simulink model "robot_4DOF"  (Simulink 7.3)
settings: Solver=ode45  StartTime=0.0  StopTime=10.0  RelTol=1e-3
libraries: dspinverses x1
settings Model: Creator=arash  LastModifiedBy=arash  TunableVars=I1,I2,I3,I4,Ixx1,Ixx2,Ixx3,Ixx4,Iyy1,Iyy2,Iyy3,Iyy4,Izz1,Izz2,Izz3,Izz4,Kd,Ki,Kp,Ts,c1,c2,c3,c4,g,l1,l2,l3,l4,m1,m2,m3,m4,statesint,tauin,tout,yout  TunableVarsStorageClass=Auto,Auto,Auto,Auto,Auto,Auto,Auto,Auto,Auto,Auto,Auto,Auto,Auto,Auto,Auto,Auto,Auto,Auto,Auto,Auto,Auto,Auto,Auto,Auto,Auto,Auto,Auto,Auto,Auto,Auto,Auto,Auto,Auto,Auto,Auto,Auto,Auto  TunableVarsTypeQualifier=,,,,,,,,,,,,,,,,,,,,,,,,,,,,,,,,,,,,
settings OptimizationCC: InlineParams=on

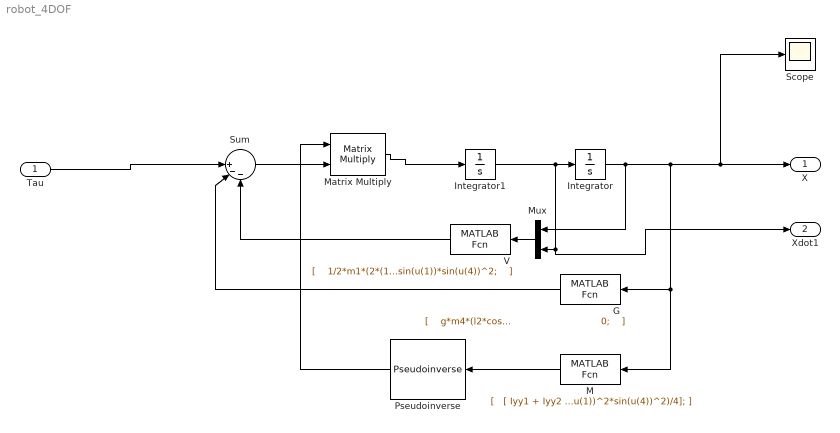
== system robot_4DOF ==
  Tau : Inport  OutDataType=fixdt(1, 16)  OutScaling=2^0
  G : MATLABFcn  MATLABFcn=|  OutputDimensions=4  OutputSignalType=real  Output1D=off
      | [
      |  
      |  g*m4*(l2*cos(u(1) + u(2)) + l1*cos(u(1)) + 1/2*l3*cos(u(1) + u(2) + u(3))) + g*m3*(1/2*l2*cos(u(1) + u(2)) + l1*cos(u(1))) + 1/2*g*l1*m2*cos(u(1));
      |                                                          g*m4*(l2*cos(u(1) + u(2)) + 1/2*l3*cos(u(1) + u(2) + u(3))) + 1/2*g*l2*m3*cos(u(1) + u(2));
      |                                                                                                                 1/2*g*l3*m4*cos(u(1) + u(2) + u(3));
      |                                                                                                                                                   0;
      |  
      |  ]
  Integrator : Integrator
  Integrator1 : Integrator
  M : MATLABFcn  MATLABFcn=|  OutputDimensions=[4 4]  OutputSignalType=real  Output1D=off
      | [
      |  
      | [ Iyy1 + Iyy2 + 1.0*Iyy3 + (m3*(2*(1.0*l2*sin(u(1) + u(2)) + l1*sin(u(1)) + 0.5*l3*sin(u(1) + u(2) + u(3)))*(l2*sin(u(1) + u(2)) + l1*sin(u(1)) + (l3*sin(u(1) + u(2) + u(3)))/2)*cos(u(4))^2 + 2*(1.0*l2*sin(u(1) + u(2)) + l1*sin(u(1)) + 0.5*l3*sin(u(1) + u(2) + u(3)))*(l2*sin(u(1) + u(2)) + l1*sin(u(1)) + (l3*sin(u(1) + u(2) + u(3)))/2)*sin(u(4))^2 + 2*(l2*cos(u(1) + u(2)) + l1*cos(u(1)) + (l3*cos(u(1) + u(2) + u(3)))/2)*(1.0*l2*cos(u(1) + u(2)) + l1*cos(u(1)) + 0.5*l3*cos(u(1) + u(2) + u(3)))))/2 + (l1^2*m1)/4 + (m2*(2*((l2*sin(u(1) + u(2)))/2 + l1*sin(u(1)))*(0.5*l2*sin(u(1) + u(2)) + l1*sin(u(1)))*cos(u(4))^2 + 2*((l2*sin(u(1) + u(2)))/2 + l1*sin(u(1)))*(0.5*l2*sin(u(1) + u(2)) + l1*sin(u(1)))*sin(u(4))^2 + 2*((l2*cos(u(1) + u(2)))/2 + l1*cos(u(1)))*(0.5*l2*cos(u(1) + u(2)) + l1*cos(u(1)))))/2, Iyy2 + 1.0*Iyy3 + (m3*(2*(1.0*l2*sin(u(1) + u(2)) + 0.5*l3*sin(u(1) + u(2) + u(3)))*(l2*sin(u(1) + u(2)) + l1*sin(u(1)) + (l3*sin(u(1) + u(2) + u(3)))/2)*cos(u(4))^2 + 2*(1.0*l2*sin(u(1) + u(2)) + 0.5*l3*sin(u(1) + u(2) + u(3)))*(l2*sin(u(1) + u(2)) + l1*sin(u(1)) + (l3*sin(u(1) + u(2) + u(3)))/2)*sin(u(4))^2 + 2*(1.0*l2*cos(u(1) + u(2)) + 0.5*l3*cos(u(1) + u(2) + u(3)))*(l2*cos(u(1) + u(2)) + l1*cos(u(1)) + (l3*cos(u(1) + u(2) + u(3)))/2)))/2 + (m2*(1.0*l2*sin(u(1) + u(2))*((l2*sin(u(1) + u(2)))/2 + l1*sin(u(1)))*cos(u(4))^2 + 1.0*l2*sin(u(1) + u(2))*((l2*sin(u(1) + u(2)))/2 + l1*sin(u(1)))*sin(u(4))^2 + 1.0*l2*cos(u(1) + u(2))*((l2*cos(u(1) + u(2)))/2 + l1*cos(u(1)))))/2, 1.0*Iyy3 + (m3*(1.0*l3*sin(u(1) + u(2) + u(3))*(l2*sin(u(1) + u(2)) + l1*sin(u(1)) + (l3*sin(u(1) + u(2) + u(3)))/2)*cos(u(4))^2 + 1.0*l3*sin(u(1) + u(2) + u(3))*(l2*sin(u(1) + u(2)) + l1*sin(u(1)) + (l3*sin(u(1) + u(2) + u(3)))/2)*sin(u(4))^2 + 1.0*l3*cos(u(1) + u(2) + u(3))*(l2*cos(u(1) + u(2)) + l1*cos(u(1)) + (l3*cos(u(1) + u(2) + u(3)))/2)))/2,                                                                                                                                                                                                                                                                                                                                                                                                                                                                                                                                                                                    0];
      | [                                                                                                                                                                                                                                                                                                                                                                                                                                                                                                                                                                                                                                                                                 Iyy2 + Iyy3 + (l2^2*m2)/4 + l2^2*m3 + (l3^2*m3)/4 + (l1*l3*m3*cos(u(2) + u(3)))/2 + (l1*l2*m2*cos(u(2)))/2 + l1*l2*m3*cos(u(2)) + l2*l3*m3*cos(u(3)),                                                                                                                                                                                                                                                                                                                                                                                                                                                                                                                                                                                                                                    Iyy2 + Iyy3 + (l2^2*m2)/4 + l2^2*m3 + (l3^2*m3)/4 + l2*l3*m3*cos(u(3)),                                                                                                                                                                                                                                                                                                                    (m3*l3^2)/4 + (l2*m3*cos(u(3))*l3)/2 + Iyy3,                                                                                                                                                                                                                                                                                                                                                                                                                                                                                                                                                                                    0];
      | [                                                                                                                                                                                                                                                                                                                                                                                                                                                                                                                                                                                                                                                                                                                                                          Iyy3 + (l3^2*m3)/4 + (l1*l3*m3*cos(u(2) + u(3)))/2 + (l2*l3*m3*cos(u(3)))/2,                                                                                                                                                                                                                                                                                                                                                                                                                                                                                                                                                                                                                                                               (m3*l3^2)/4 + (l2*m3*cos(u(3))*l3)/2 + Iyy3,                                                                                                                                                                                                                                                                                                                                             (m3*l3^2)/4 + Iyy3,                                                                                                                                                                                                                                                                                                                                                                                                                                                                                                                                                                                    0];
      | [                                                                                                                                                                                                                                                                                                                                                                                                                                                                                                                                                                                                                                                                                                                                                                                                                                    0,                                                                                                                                                                                                                                                                                                                                                                                                                                                                                                                                                                                                                                                                                                         0,                                                                                                                                                                                                                                                                                                                                                              0, I4 - Izz2*(cos(u(1) + u(2))^2 - 1) + (m2*(2*cos(u(4))^2*((l2*cos(u(1) + u(2)))/2 + l1*cos(u(1)))^2 + 2*sin(u(4))^2*((l2*cos(u(1) + u(2)))/2 + l1*cos(u(1)))^2))/2 + Ixx3*cos(u(1) + u(2) + u(3))^2 - Izz1*(cos(u(1))^2 - 1) - Izz3*(cos(u(1) + u(2) + u(3))^2 - 1) + Ixx2*cos(u(1) + u(2))^2 + Ixx1*cos(u(1))^2 + (m3*(2*cos(u(4))^2*(l2*cos(u(1) + u(2)) + l1*cos(u(1)) + (l3*cos(u(1) + u(2) + u(3)))/2)^2 + 2*sin(u(4))^2*(l2*cos(u(1) + u(2)) + l1*cos(u(1)) + (l3*cos(u(1) + u(2) + u(3)))/2)^2))/2 + (l1^2*m1*cos(u(1))^2*cos(u(4))^2)/4 + (l1^2*m1*cos(u(1))^2*sin(u(4))^2)/4];
      | ]
  Matrix Multiply : Product  Multiplication=Matrix(*)  OutDataType=sfix(16)  OutScaling=2^0
  Mux : Mux  Inputs=2
  Pseudoinverse : dspinverses/Pseudoinverse  wanterr=off
  Scope : Scope
      settings: YMin=-2.75  YMax=0.25
  Sum : Sum  Inputs=||+--  OutDataType=fixdt(1, 16)  OutScaling=2^0
  V : MATLABFcn  MATLABFcn=|  OutputDimensions=4  OutputSignalType=real  Output1D=off
      | [
      |  
      |  1/2*m1*(2*(1/2*l1*u(8)*sin(u(1))*sin(u(4)) - 1/2*l1*u(5)*cos(u(1))*cos(u(4)))*(1/2*l1*u(5)*cos(u(4))*sin(u(1)) + 1/2*l1*u(8)*cos(u(1))*sin(u(4))) - 2*(1/2*l1*u(5)*sin(u(1))*sin(u(4)) - 1/2*l1*u(8)*cos(u(1))*cos(u(4)))*(1/2*l1*u(5)*cos(u(1))*sin(u(4)) + 1/2*l1*u(8)*cos(u(4))*sin(u(1))) + 1/2*l1^2*u(5)^2*cos(u(1))*sin(u(1))) + 1/2*m2*(2*sin(u(4))*(1/2*l2*sin(u(1) + u(2)) + l1*sin(u(1)))*(sin(u(4))*(1/2*l2*cos(u(1) + u(2)) + l1*cos(u(1)))*u(8)^2 + 2*cos(u(4))*(l1*u(5)*sin(u(1)) + 1/2*l2*sin(u(1) + u(2))*(u(5) + u(6)))*u(8) + sin(u(4))*(1/2*l2*cos(u(1) + u(2))*(u(5) + u(6))^2 + l1*u(5)^2*cos(u(1)))) - 2*(1/2*l2*sin(u(1) + u(2))*(u(5) + u(6))^2 + l1*u(5)^2*sin(u(1)))*(1/2*l2*cos(u(1) + u(2)) + l1*cos(u(1))) - 2*(l1*u(5)*cos(u(1)) + 1/2*l2*cos(u(1) + u(2))*(u(5) + u(6)))*(l1*u(5)*sin(u(1)) + 1/2*l2*sin(u(1) + u(2))*(u(5) + u(6))) + 2*cos(u(4))*(cos(u(4))*(l1*u(5)*sin(u(1)) + 1/2*l2*sin(u(1) + u(2))*(u(5) + u(6))) + u(8)*sin(u(4))*(1/2*l2*cos(u(1) + u(2)) + l1*cos(u(1))))*(l1*u(5)*cos(u(1)) + 1/2*l2*cos(u(1) + u(2))*(u(5) + u(6))) + 2*sin(u(4))*(sin(u(4))*(l1*u(5)*sin(u(1)) + 1/2*l2*sin(u(1) + u(2))*(u(5) + u(6))) - u(8)*cos(u(4))*(1/2*l2*cos(u(1) + u(2)) + l1*cos(u(1))))*(l1*u(5)*cos(u(1)) + 1/2*l2*cos(u(1) + u(2))*(u(5) + u(6))) + 2*cos(u(4))*(1/2*l2*sin(u(1) + u(2)) + l1*sin(u(1)))*(cos(u(4))*(1/2*l2*cos(u(1) + u(2)) + l1*cos(u(1)))*u(8)^2 - 2*sin(u(4))*(l1*u(5)*sin(u(1)) + 1/2*l2*sin(u(1) + u(2))*(u(5) + u(6)))*u(8) + cos(u(4))*(1/2*l2*cos(u(1) + u(2))*(u(5) + u(6))^2 + l1*u(5)^2*cos(u(1)))) + 2*u(8)*cos(u(4))*(sin(u(4))*(l1*u(5)*sin(u(1)) + 1/2*l2*sin(u(1) + u(2))*(u(5) + u(6))) - u(8)*cos(u(4))*(1/2*l2*cos(u(1) + u(2)) + l1*cos(u(1))))*(1/2*l2*sin(u(1) + u(2)) + l1*sin(u(1))) - 2*u(8)*sin(u(4))*(cos(u(4))*(l1*u(5)*sin(u(1)) + 1/2*l2*sin(u(1) + u(2))*(u(5) + u(6))) + u(8)*sin(u(4))*(1/2*l2*cos(u(1) + u(2)) + l1*cos(u(1))))*(1/2*l2*sin(u(1) + u(2)) + l1*sin(u(1)))) + c1*u(5) - 1/2*m3*(2*(sin(u(4))*(l1*u(5)*cos(u(1)) + 1/2*l3*cos(u(1) + u(2) + u(3))*(u(5) + u(6) + u(7)) + l2*cos(u(1) + u(2))*(u(5) + u(6))) + u(8)*cos(u(4))*(l2*sin(u(1) + u(2)) + l1*sin(u(1)) + 1/2*l3*sin(u(1) + u(2) + u(3))))*(sin(u(4))*(l1*u(5)*sin(u(1)) + 1/2*l3*sin(u(1) + u(2) + u(3))*(u(5) + u(6) + u(7)) + l2*sin(u(1) + u(2))*(u(5) + u(6))) - u(8)*cos(u(4))*(l2*cos(u(1) + u(2)) + l1*cos(u(1)) + 1/2*l3*cos(u(1) + u(2) + u(3)))) - 2*(l1*u(5)*sin(u(1)) + 1/2*l3*sin(u(1) + u(2) + u(3))*(u(5) + u(6) + u(7)) + l2*sin(u(1) + u(2))*(u(5) + u(6)))*(l1*u(5)*cos(u(1)) + 1/2*l3*cos(u(1) + u(2) + u(3))*(u(5) + u(6) + u(7)) + l2*cos(u(1) + u(2))*(u(5) + u(6))) + 2*(cos(u(4))*(l1*u(5)*sin(u(1)) + 1/2*l3*sin(u(1) + u(2) + u(3))*(u(5) + u(6) + u(7)) + l2*sin(u(1) + u(2))*(u(5) + u(6))) + u(8)*sin(u(4))*(l2*cos(u(1) + u(2)) + l1*cos(u(1)) + 1/2*l3*cos(u(1) + u(2) + u(3))))*(cos(u(4))*(l1*u(5)*cos(u(1)) + 1/2*l3*cos(u(1) + u(2) + u(3))*(u(5) + u(6) + u(7)) + l2*cos(u(1) + u(2))*(u(5) + u(6))) - u(8)*sin(u(4))*(l2*sin(u(1) + u(2)) + l1*sin(u(1)) + 1/2*l3*sin(u(1) + u(2) + u(3))))) - 1/2*m2*(2*(sin(u(4))*(l1*u(5)*cos(u(1)) + 1/2*l2*cos(u(1) + u(2))*(u(5) + u(6))) + u(8)*cos(u(4))*(1/2*l2*sin(u(1) + u(2)) + l1*sin(u(1))))*(sin(u(4))*(l1*u(5)*sin(u(1)) + 1/2*l2*sin(u(1) + u(2))*(u(5) + u(6))) - u(8)*cos(u(4))*(1/2*l2*cos(u(1) + u(2)) + l1*cos(u(1)))) + 2*(cos(u(4))*(l1*u(5)*sin(u(1)) + 1/2*l2*sin(u(1) + u(2))*(u(5) + u(6))) + u(8)*sin(u(4))*(1/2*l2*cos(u(1) + u(2)) + l1*cos(u(1))))*(cos(u(4))*(l1*u(5)*cos(u(1)) + 1/2*l2*cos(u(1) + u(2))*(u(5) + u(6))) - u(8)*sin(u(4))*(1/2*l2*sin(u(1) + u(2)) + l1*sin(u(1)))) - 2*(l1*u(5)*cos(u(1)) + 1/2*l2*cos(u(1) + u(2))*(u(5) + u(6)))*(l1*u(5)*sin(u(1)) + 1/2*l2*sin(u(1) + u(2))*(u(5) + u(6)))) + 1/2*m3*(2*cos(u(4))*(l2*sin(u(1) + u(2)) + l1*sin(u(1)) + 1/2*l3*sin(u(1) + u(2) + u(3)))*(cos(u(4))*(l2*cos(u(1) + u(2)) + l1*cos(u(1)) + 1/2*l3*cos(u(1) + u(2) + u(3)))*u(8)^2 - 2*sin(u(4))*(l1*u(5)*sin(u(1)) + 1/2*l3*sin(u(1) + u(2) + u(3))*(u(5) + u(6) + u(7)) + l2*sin(u(1) + u(2))*(u(5) + u(6)))*u(8) + cos(u(4))*(1/2*l3*cos(u(1) + u(2) + u(3))*(u(5) + u(6) + u(7))^2 + l2*cos(u(1) + u(2))*(u(5) + u(6))^2 + l1*u(5)^2*cos(u(1)))) - 2*(1/2*l3*sin(u(1) + u(2) + u(3))*(u(5) + u(6) + u(7))^2 + l2*sin(u(1) + u(2))*(u(5) + u(6))^2 + l1*u(5)^2*sin(u(1)))*(l2*cos(u(1) + u(2)) + l1*cos(u(1)) + 1/2*l3*cos(u(1) + u(2) + u(3))) - 2*(l1*u(5)*sin(u(1)) + 1/2*l3*sin(u(1) + u(2) + u(3))*(u(5) + u(6) + u(7)) + l2*sin(u(1) + u(2))*(u(5) + u(6)))*(l1*u(5)*cos(u(1)) + 1/2*l3*cos(u(1) + u(2) + u(3))*(u(5) + u(6) + u(7)) + l2*cos(u(1) + u(2))*(u(5) + u(6))) + 2*sin(u(4))*(l2*sin(u(1) + u(2)) + l1*sin(u(1)) + 1/2*l3*sin(u(1) + u(2) + u(3)))*(sin(u(4))*(l2*cos(u(1) + u(2)) + l1*cos(u(1)) + 1/2*l3*cos(u(1) + u(2) + u(3)))*u(8)^2 + 2*cos(u(4))*(l1*u(5)*sin(u(1)) + 1/2*l3*sin(u(1) + u(2) + u(3))*(u(5) + u(6) + u(7)) + l2*sin(u(1) + u(2))*(u(5) + u(6)))*u(8) + sin(u(4))*(1/2*l3*cos(u(1) + u(2) + u(3))*(u(5) + u(6) + u(7))^2 + l2*cos(u(1) + u(2))*(u(5) + u(6))^2 + l1*u(5)^2*cos(u(1)))) + 2*cos(u(4))*(cos(u(4))*(l1*u(5)*sin(u(1)) + 1/2*l3*sin(u(1) + u(2) + u(3))*(u(5) + u(6) + u(7)) + l2*sin(u(1) + u(2))*(u(5) + u(6))) + u(8)*sin(u(4))*(l2*cos(u(1) + u(2)) + l1*cos(u(1)) + 1/2*l3*cos(u(1) + u(2) + u(3))))*(l1*u(5)*cos(u(1)) + 1/2*l3*cos(u(1) + u(2) + u(3))*(u(5) + u(6) + u(7)) + l2*cos(u(1) + u(2))*(u(5) + u(6))) + 2*sin(u(4))*(sin(u(4))*(l1*u(5)*sin(u(1)) + 1/2*l3*sin(u(1) + u(2) + u(3))*(u(5) + u(6) + u(7)) + l2*sin(u(1) + u(2))*(u(5) + u(6))) - u(8)*cos(u(4))*(l2*cos(u(1) + u(2)) + l1*cos(u(1)) + 1/2*l3*cos(u(1) + u(2) + u(3))))*(l1*u(5)*cos(u(1)) + 1/2*l3*cos(u(1) + u(2) + u(3))*(u(5) + u(6) + u(7)) + l2*cos(u(1) + u(2))*(u(5) + u(6))) + 2*u(8)*cos(u(4))*(sin(u(4))*(l1*u(5)*sin(u(1)) + 1/2*l3*sin(u(1) + u(2) + u(3))*(u(5) + u(6) + u(7)) + l2*sin(u(1) + u(2))*(u(5) + u(6))) - u(8)*cos(u(4))*(l2*cos(u(1) + u(2)) + l1*cos(u(1)) + 1/2*l3*cos(u(1) + u(2) + u(3))))*(l2*sin(u(1) + u(2)) + l1*sin(u(1)) + 1/2*l3*sin(u(1) + u(2) + u(3))) - 2*u(8)*sin(u(4))*(cos(u(4))*(l1*u(5)*sin(u(1)) + 1/2*l3*sin(u(1) + u(2) + u(3))*(u(5) + u(6) + u(7)) + l2*sin(u(1) + u(2))*(u(5) + u(6))) + u(8)*sin(u(4))*(l2*cos(u(1) + u(2)) + l1*cos(u(1)) + 1/2*l3*cos(u(1) + u(2) + u(3))))*(l2*sin(u(1) + u(2)) + l1*sin(u(1)) + 1/2*l3*sin(u(1) + u(2) + u(3)))) + Ixx1*u(8)^2*cos(u(1))*sin(u(1)) - Izz1*u(8)^2*cos(u(1))*sin(u(1)) + Ixx3*u(8)^2*cos(u(1) + u(2) + u(3))*sin(u(1) + u(2) + u(3)) - Izz3*u(8)^2*cos(u(1) + u(2) + u(3))*sin(u(1) + u(2) + u(3)) + Ixx2*u(8)^2*cos(u(1) + u(2))*sin(u(1) + u(2)) - Izz2*u(8)^2*cos(u(1) + u(2))*sin(u(1) + u(2));
      |                                                                                                                                                                                                                                                                                                                                                                                                                                                                                                                                                                                                                                                                                                                                                                                                                                                                                                                                                                                                                                                                                                                                                                                                                                                                                                                                                                                                                                                                                                                                                                                                                                                                                                                                                                                                                                                                                                                                                                                                                                                                                                                                                                                                                                                                                                                                                                                                                                                                                                                                                                                                                                                                                                                                                                                                                                                                                                                                                                                                                                                                                                                                                                                                                                                                                                                                                                                                                                                                                                                                                                                                                                                                                                                                                                                                                                                                                                                                                                                                                                                                                                                                                                                                                                                                                                                                                                                                                                                                                                                                                                                                                                                                                                                                                                                                                                                                                                                                                                                                                                                                                       c2*u(6) - 1/2*m3*(2*(cos(u(4))*(l1*u(5)*sin(u(1)) + 1/2*l3*sin(u(1) + u(2) + u(3))*(u(5) + u(6) + u(7)) + l2*sin(u(1) + u(2))*(u(5) + u(6))) + u(8)*sin(u(4))*(l2*cos(u(1) + u(2)) + l1*cos(u(1)) + 1/2*l3*cos(u(1) + u(2) + u(3))))*(cos(u(4))*(1/2*l3*cos(u(1) + u(2) + u(3))*(u(5) + u(6) + u(7)) + l2*cos(u(1) + u(2))*(u(5) + u(6))) - u(8)*sin(u(4))*(l2*sin(u(1) + u(2)) + 1/2*l3*sin(u(1) + u(2) + u(3)))) + 2*(sin(u(4))*(l1*u(5)*sin(u(1)) + 1/2*l3*sin(u(1) + u(2) + u(3))*(u(5) + u(6) + u(7)) + l2*sin(u(1) + u(2))*(u(5) + u(6))) - u(8)*cos(u(4))*(l2*cos(u(1) + u(2)) + l1*cos(u(1)) + 1/2*l3*cos(u(1) + u(2) + u(3))))*(sin(u(4))*(1/2*l3*cos(u(1) + u(2) + u(3))*(u(5) + u(6) + u(7)) + l2*cos(u(1) + u(2))*(u(5) + u(6))) + u(8)*cos(u(4))*(l2*sin(u(1) + u(2)) + 1/2*l3*sin(u(1) + u(2) + u(3)))) - 2*(1/2*l3*sin(u(1) + u(2) + u(3))*(u(5) + u(6) + u(7)) + l2*sin(u(1) + u(2))*(u(5) + u(6)))*(l1*u(5)*cos(u(1)) + 1/2*l3*cos(u(1) + u(2) + u(3))*(u(5) + u(6) + u(7)) + l2*cos(u(1) + u(2))*(u(5) + u(6)))) - 1/2*m2*(2*(cos(u(4))*(l1*u(5)*sin(u(1)) + 1/2*l2*sin(u(1) + u(2))*(u(5) + u(6))) + u(8)*sin(u(4))*(1/2*l2*cos(u(1) + u(2)) + l1*cos(u(1))))*(1/2*l2*cos(u(1) + u(2))*cos(u(4))*(u(5) + u(6)) - 1/2*l2*u(8)*sin(u(1) + u(2))*sin(u(4))) + 2*(sin(u(4))*(l1*u(5)*sin(u(1)) + 1/2*l2*sin(u(1) + u(2))*(u(5) + u(6))) - u(8)*cos(u(4))*(1/2*l2*cos(u(1) + u(2)) + l1*cos(u(1))))*(1/2*l2*cos(u(1) + u(2))*sin(u(4))*(u(5) + u(6)) + 1/2*l2*u(8)*sin(u(1) + u(2))*cos(u(4))) - l2*sin(u(1) + u(2))*(l1*u(5)*cos(u(1)) + 1/2*l2*cos(u(1) + u(2))*(u(5) + u(6)))*(u(5) + u(6))) + Ixx3*u(8)^2*cos(u(1) + u(2) + u(3))*sin(u(1) + u(2) + u(3)) - Izz3*u(8)^2*cos(u(1) + u(2) + u(3))*sin(u(1) + u(2) + u(3)) + Ixx2*u(8)^2*cos(u(1) + u(2))*sin(u(1) + u(2)) - Izz2*u(8)^2*cos(u(1) + u(2))*sin(u(1) + u(2)) - 1/2*l2*l3*m3*u(7)^2*sin(u(3)) - 1/2*l1*l3*m3*u(5)*u(6)*sin(u(2) + u(3)) - 1/2*l1*l3*m3*u(5)*u(7)*sin(u(2) + u(3)) - 1/2*l1*l2*m2*u(5)*u(6)*sin(u(2)) - l1*l2*m3*u(5)*u(6)*sin(u(2)) - l2*l3*m3*u(5)*u(7)*sin(u(3)) - l2*l3*m3*u(6)*u(7)*sin(u(3));
      |                                                                                                                                                                                                                                                                                                                                                                                                                                                                                                                                                                                                                                                                                                                                                                                                                                                                                                                                                                                                                                                                                                                                                                                                                                                                                                                                                                                                                                                                                                                                                                                                                                                                                                                                                                                                                                                                                                                                                                                                                                                                                                                                                                                                                                                                                                                                                                                                                                                                                                                                                                                                                                                                                                                                                                                                                                                                                                                                                                                                                                                                                                                                                                                                                                                                                                                                                                                                                                                                                                                                                                                                                                                                                                                                                                                                                                                                                                                                                                                                                                                                                                                                                                                                                                                                                                                                                                                                                                                                                                                                                                                                                                                                                                                                                                                                                                                                                                                                                                                                                                                                                                                                                                                                                                                                                                                                                                                                                                                                                                                                                                                                                                                                                                                                                                                                                                                                                                                                                                                                                                                                                                                                    c3*u(7) + 1/2*m3*(2*(1/2*l3*u(8)*sin(u(1) + u(2) + u(3))*sin(u(4)) - 1/2*l3*cos(u(1) + u(2) + u(3))*cos(u(4))*(u(5) + u(6) + u(7)))*(cos(u(4))*(l1*u(5)*sin(u(1)) + 1/2*l3*sin(u(1) + u(2) + u(3))*(u(5) + u(6) + u(7)) + l2*sin(u(1) + u(2))*(u(5) + u(6))) + u(8)*sin(u(4))*(l2*cos(u(1) + u(2)) + l1*cos(u(1)) + 1/2*l3*cos(u(1) + u(2) + u(3)))) - 2*(1/2*l3*u(8)*sin(u(1) + u(2) + u(3))*cos(u(4)) + 1/2*l3*cos(u(1) + u(2) + u(3))*sin(u(4))*(u(5) + u(6) + u(7)))*(sin(u(4))*(l1*u(5)*sin(u(1)) + 1/2*l3*sin(u(1) + u(2) + u(3))*(u(5) + u(6) + u(7)) + l2*sin(u(1) + u(2))*(u(5) + u(6))) - u(8)*cos(u(4))*(l2*cos(u(1) + u(2)) + l1*cos(u(1)) + 1/2*l3*cos(u(1) + u(2) + u(3)))) + l3*sin(u(1) + u(2) + u(3))*(u(5) + u(6) + u(7))*(l1*u(5)*cos(u(1)) + 1/2*l3*cos(u(1) + u(2) + u(3))*(u(5) + u(6) + u(7)) + l2*cos(u(1) + u(2))*(u(5) + u(6)))) + Ixx3*u(8)^2*cos(u(1) + u(2) + u(3))*sin(u(1) + u(2) + u(3)) - Izz3*u(8)^2*cos(u(1) + u(2) + u(3))*sin(u(1) + u(2) + u(3)) - 1/2*l1*l3*m3*u(5)*u(6)*sin(u(2) + u(3)) - 1/2*l1*l3*m3*u(5)*u(7)*sin(u(2) + u(3)) - 1/2*l2*l3*m3*u(5)*u(7)*sin(u(3)) - 1/2*l2*l3*m3*u(6)*u(7)*sin(u(3));
      |                                                                                                                                                                                                                                                                                                                                                                                                                                                                                                                                                                                                                                                                                                                                                                                                                                                                                                                                                                                                                                                                                                                                                                                                                                                                                                                                                                                                                                                                                                                                                                                                                                                                                                                                                                                                                                                                                                                                                                                                                                                                                                                                                                                                                                                                                                                                                                                                                                                                                                                                                                                                                                                                                                                                                                                                                                                                                1/2*m2*(2*cos(u(4))*(sin(u(4))*(l1*u(5)*sin(u(1)) + 1/2*l2*sin(u(1) + u(2))*(u(5) + u(6))) - u(8)*cos(u(4))*(1/2*l2*cos(u(1) + u(2)) + l1*cos(u(1))))*(l1*u(5)*sin(u(1)) + 1/2*l2*sin(u(1) + u(2))*(u(5) + u(6))) - 2*sin(u(4))*(cos(u(4))*(l1*u(5)*sin(u(1)) + 1/2*l2*sin(u(1) + u(2))*(u(5) + u(6))) + u(8)*sin(u(4))*(1/2*l2*cos(u(1) + u(2)) + l1*cos(u(1))))*(l1*u(5)*sin(u(1)) + 1/2*l2*sin(u(1) + u(2))*(u(5) + u(6))) - 2*cos(u(4))*(1/2*l2*cos(u(1) + u(2)) + l1*cos(u(1)))*(sin(u(4))*(1/2*l2*cos(u(1) + u(2)) + l1*cos(u(1)))*u(8)^2 + 2*cos(u(4))*(l1*u(5)*sin(u(1)) + 1/2*l2*sin(u(1) + u(2))*(u(5) + u(6)))*u(8) + sin(u(4))*(1/2*l2*cos(u(1) + u(2))*(u(5) + u(6))^2 + l1*u(5)^2*cos(u(1)))) + 2*sin(u(4))*(1/2*l2*cos(u(1) + u(2)) + l1*cos(u(1)))*(cos(u(4))*(1/2*l2*cos(u(1) + u(2)) + l1*cos(u(1)))*u(8)^2 - 2*sin(u(4))*(l1*u(5)*sin(u(1)) + 1/2*l2*sin(u(1) + u(2))*(u(5) + u(6)))*u(8) + cos(u(4))*(1/2*l2*cos(u(1) + u(2))*(u(5) + u(6))^2 + l1*u(5)^2*cos(u(1)))) + 2*u(8)*cos(u(4))*(cos(u(4))*(l1*u(5)*sin(u(1)) + 1/2*l2*sin(u(1) + u(2))*(u(5) + u(6))) + u(8)*sin(u(4))*(1/2*l2*cos(u(1) + u(2)) + l1*cos(u(1))))*(1/2*l2*cos(u(1) + u(2)) + l1*cos(u(1))) + 2*u(8)*sin(u(4))*(sin(u(4))*(l1*u(5)*sin(u(1)) + 1/2*l2*sin(u(1) + u(2))*(u(5) + u(6))) - u(8)*cos(u(4))*(1/2*l2*cos(u(1) + u(2)) + l1*cos(u(1))))*(1/2*l2*cos(u(1) + u(2)) + l1*cos(u(1)))) + 1/2*m3*(2*cos(u(4))*(sin(u(4))*(l1*u(5)*sin(u(1)) + 1/2*l3*sin(u(1) + u(2) + u(3))*(u(5) + u(6) + u(7)) + l2*sin(u(1) + u(2))*(u(5) + u(6))) - u(8)*cos(u(4))*(l2*cos(u(1) + u(2)) + l1*cos(u(1)) + 1/2*l3*cos(u(1) + u(2) + u(3))))*(l1*u(5)*sin(u(1)) + 1/2*l3*sin(u(1) + u(2) + u(3))*(u(5) + u(6) + u(7)) + l2*sin(u(1) + u(2))*(u(5) + u(6))) - 2*sin(u(4))*(cos(u(4))*(l1*u(5)*sin(u(1)) + 1/2*l3*sin(u(1) + u(2) + u(3))*(u(5) + u(6) + u(7)) + l2*sin(u(1) + u(2))*(u(5) + u(6))) + u(8)*sin(u(4))*(l2*cos(u(1) + u(2)) + l1*cos(u(1)) + 1/2*l3*cos(u(1) + u(2) + u(3))))*(l1*u(5)*sin(u(1)) + 1/2*l3*sin(u(1) + u(2) + u(3))*(u(5) + u(6) + u(7)) + l2*sin(u(1) + u(2))*(u(5) + u(6))) - 2*cos(u(4))*(l2*cos(u(1) + u(2)) + l1*cos(u(1)) + 1/2*l3*cos(u(1) + u(2) + u(3)))*(sin(u(4))*(l2*cos(u(1) + u(2)) + l1*cos(u(1)) + 1/2*l3*cos(u(1) + u(2) + u(3)))*u(8)^2 + 2*cos(u(4))*(l1*u(5)*sin(u(1)) + 1/2*l3*sin(u(1) + u(2) + u(3))*(u(5) + u(6) + u(7)) + l2*sin(u(1) + u(2))*(u(5) + u(6)))*u(8) + sin(u(4))*(1/2*l3*cos(u(1) + u(2) + u(3))*(u(5) + u(6) + u(7))^2 + l2*cos(u(1) + u(2))*(u(5) + u(6))^2 + l1*u(5)^2*cos(u(1)))) + 2*sin(u(4))*(l2*cos(u(1) + u(2)) + l1*cos(u(1)) + 1/2*l3*cos(u(1) + u(2) + u(3)))*(cos(u(4))*(l2*cos(u(1) + u(2)) + l1*cos(u(1)) + 1/2*l3*cos(u(1) + u(2) + u(3)))*u(8)^2 - 2*sin(u(4))*(l1*u(5)*sin(u(1)) + 1/2*l3*sin(u(1) + u(2) + u(3))*(u(5) + u(6) + u(7)) + l2*sin(u(1) + u(2))*(u(5) + u(6)))*u(8) + cos(u(4))*(1/2*l3*cos(u(1) + u(2) + u(3))*(u(5) + u(6) + u(7))^2 + l2*cos(u(1) + u(2))*(u(5) + u(6))^2 + l1*u(5)^2*cos(u(1)))) + 2*u(8)*cos(u(4))*(cos(u(4))*(l1*u(5)*sin(u(1)) + 1/2*l3*sin(u(1) + u(2) + u(3))*(u(5) + u(6) + u(7)) + l2*sin(u(1) + u(2))*(u(5) + u(6))) + u(8)*sin(u(4))*(l2*cos(u(1) + u(2)) + l1*cos(u(1)) + 1/2*l3*cos(u(1) + u(2) + u(3))))*(l2*cos(u(1) + u(2)) + l1*cos(u(1)) + 1/2*l3*cos(u(1) + u(2) + u(3))) + 2*u(8)*sin(u(4))*(sin(u(4))*(l1*u(5)*sin(u(1)) + 1/2*l3*sin(u(1) + u(2) + u(3))*(u(5) + u(6) + u(7)) + l2*sin(u(1) + u(2))*(u(5) + u(6))) - u(8)*cos(u(4))*(l2*cos(u(1) + u(2)) + l1*cos(u(1)) + 1/2*l3*cos(u(1) + u(2) + u(3))))*(l2*cos(u(1) + u(2)) + l1*cos(u(1)) + 1/2*l3*cos(u(1) + u(2) + u(3)))) + c4*u(8) - 2*Ixx3*u(8)*cos(u(1) + u(2) + u(3))*sin(u(1) + u(2) + u(3))*(u(5) + u(6) + u(7)) + 2*Izz3*u(8)*cos(u(1) + u(2) + u(3))*sin(u(1) + u(2) + u(3))*(u(5) + u(6) + u(7)) - 2*Ixx1*u(5)*u(8)*cos(u(1))*sin(u(1)) + 2*Izz1*u(5)*u(8)*cos(u(1))*sin(u(1)) - 2*Ixx2*u(8)*cos(u(1) + u(2))*sin(u(1) + u(2))*(u(5) + u(6)) + 2*Izz2*u(8)*cos(u(1) + u(2))*sin(u(1) + u(2))*(u(5) + u(6)) - 1/2*l1^2*m1*u(5)*u(8)*cos(u(1))*cos(u(4))^2*sin(u(1)) - 1/2*l1^2*m1*u(5)*u(8)*cos(u(1))*sin(u(1))*sin(u(4))^2;
      |  
      |  ]
  X : Outport  OutDataType=fixdt(1, 16)  OutScaling=2^0
  Xdot1 : Outport  Port=2  OutDataType=fixdt(1, 16)  OutScaling=2^0
  wires:
  Integrator/1 -> Mux/1, G/1, M/1, X/1, Scope/1
  Integrator1/1 -> Integrator/1, Mux/2, Xdot1/1
  Mux/1 -> V/1
  M/1 -> Pseudoinverse/1
  V/1 -> Sum/3
  G/1 -> Sum/2
  Sum/1 -> Matrix Multiply/2
  Matrix Multiply/1 -> Integrator1/1
  Pseudoinverse/1 -> Matrix Multiply/1
  Tau/1 -> Sum/1
